simulink model "Inputs_Cond"  (Simulink 7.9)
settings: Solver=FixedStepDiscrete  StartTime=0.0  StopTime=10  RelTol=1e-3  SampleTimeConstraint=STIndependent
PreLoadFcn:
  | Input_Conditioning_selfinit
CloseFcn:
  | rtwprivate ssgencode ModelCloseRequest ADL
settings Model: MinMaxOverflowLogging=ForceOff  Creator=fguerin  LastModifiedBy=klindqvi  CovMetricSettings=dce  CovHTMLOptions=-aTS=1 -bRG=1 -bTC=1 -hTR=0 -nFC=0 -scm=1 -bcm=1 -xEv=0  CovHtmlReporting=off  covSaveCumulativeToWorkspaceVar=off  CovSaveSingleToWorkspaceVar=off  CovModelRefEnable=off  CovExternalEMLEnable=on
settings DataIOCC: ExternalInput=[t,u]  LimitDataPoints=off  SaveOutput=off  DSMLogging=off  SaveTime=off  SignalLoggingName=logsOut
settings OptimizationCC: InlineParams=on  InlineInvariantSignals=on  EnhancedBackFolding=on  ZeroExternalMemoryAtStartup=off  ZeroInternalMemoryAtStartup=off  EfficientFloat2IntCast=on  OptimizeModelRefInitCode=on  LifeSpan=1
settings DebuggingCC: ReadBeforeWriteMsg=EnableAllAsError  WriteAfterWriteMsg=EnableAllAsError  WriteAfterReadMsg=EnableAllAsError  AlgebraicLoopMsg=error  ArtificialAlgebraicLoopMsg=error  SaveWithDisabledLinksMsg=error  SaveWithParameterizedLinksMsg=error  CheckExecutionContextPreStartOutputMsg=on  CheckExecutionContextRuntimeOutputMsg=on  BlockPriorityViolationMsg=error  SolverPrmCheckMsg=error  MultiTaskCondExecSysMsg=warning  MultiTaskRateTransMsg=warning  IntegerOverflowMsg=none  ParameterUnderflowMsg=error  ParameterPrecisionLossMsg=error  ParameterTunabilityLossMsg=error  UnderSpecifiedDataTypeMsg=warning  UnnecessaryDatatypeConvMsg=warning  VectorMatrixConversionMsg=error  SignalLabelMismatchMsg=warning  SFcnCompatibilityMsg=error  BusObjectLabelMismatch=error  RootOutportRequireBusObject=error  AssertControl=DisableAll  ModelReferenceIOMsg=error  ModelReferenceIOMismatchMessage=error  ModelReferenceCSMismatchMessage=warning  UnknownTsInhSupMsg=error  ModelReferenceDataLoggingMessage=error  ModelReferenceSymbolNameMessage=none  StrictBusMsg=ErrorOnBusTreatedAsVector
settings HardwareCC: ProdLargestAtomicInteger=Long  ProdLargestAtomicFloat=Double  ProdIntDivRoundTo=Zero  ProdEndianess=BigEndian  ProdHWDeviceType=Freescale->MPC5500
settings ModelReferenceCC: ModelReferenceNumInstancesAllowed=Single
settings SFSimCC: SimParseCustomCode=off
settings RTWCC: SystemTargetFile=ert.tlc  TemplateMakefile=ert_default_tmf  Description=Embedded Coder  GenerateReport=on  RTWVerbose=off  ProcessScript=ert_make_rtw_hook  IncludeHyperlinkInReport=on  LaunchReport=on  GenerateTraceInfo=on  GenerateTraceReport=on  GenerateTraceReportSl=on  GenerateTraceReportSf=on  GenerateTraceReportEml=on  GenerateCodeMetricsReport=on
settings MATStruct: className=rtw.pil.Bullseye  argsAllComponents=[]  excludedModels=[]  includeReferencedModels=off  includeTopModel=on  enabled=on
settings CodeAppCC: ForceParamTrailComments=on  IgnoreCustomStorageClasses=off  IgnoreTestpoints=on  MangleLength=4  InlinedPrmAccess=Macros  ReqsInCode=on
settings ERTTargetCC: CodeReplacementLibrary=ANSI_C  MultiwordLength=2048  SupportAbsoluteTime=off  SupportNonFinite=off  SupportComplex=off  PortableWordSizes=on  InlinedParameterPlacement=NonHierarchical  ERTCustomFileTemplate=example_file_process.tlc  ConvertIfToSwitch=off  SuppressUnreachableDefaultCases=off
settings ConfigComp: Description=Design Verifier Custom Configuration Component  DVMaxProcessTime=600  DVDisplayUnsatisfiableObjectives=on  DVAutomaticStubbing=off  DVOutputDir=C:\Work\Data\Pilots\P_PSA_ECoder_BenchMark_LaGarenne\source9b\deliverable\trunk\demos\VnV_example\Projects\ADL_Project/Simulink_Test_Generation/ADL_Sim  DVModelCoverageObjectives=MCDC  DVTestSuiteOptimization=CombinedObjectives  DVDataFileName=./Tests/$ModelName$_sldvdata  DVSaveHarnessModel=on  DVHarnessModelFileName=./Tests/$ModelName$_testHarness  DVModelReferenceHarness=on  DVSaveReport=on  DVReportFileName=ADL_Sim_SLDV.html

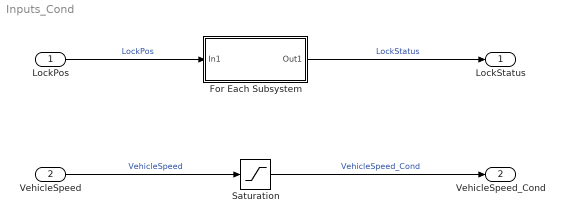
== system Inputs_Cond ==
  LockPos : Inport  OutDataTypeStr=fixdt('sfix16_Sp01')  PortDimensions=2
  VehicleSpeed : Inport  Port=2  OutDataTypeStr=single  PortDimensions=1
  For Each Subsystem : Subsystem  TreatAsAtomicUnit=on
  Saturation : Saturate  UpperLimit=350  LowerLimit=-50
  LockStatus : Outport  OutDataTypeStr=Enum: ActuatorStatus  PortDimensions=2
  VehicleSpeed_Cond : Outport  Port=2  OutDataTypeStr=single  PortDimensions=1
  wires:
  LockPos/1 -> For Each Subsystem/1(In1)  "LockPos"
  For Each Subsystem/1(Out1) -> LockStatus/1  "LockStatus"
  Saturation/1 -> VehicleSpeed_Cond/1  "VehicleSpeed_Cond"
  VehicleSpeed/1 -> Saturation/1  "VehicleSpeed"

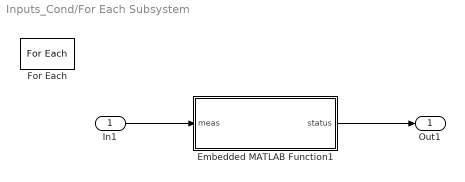
== system Inputs_Cond/For Each Subsystem ==
  In1 : Inport  Partition=on  PartitionDimension=1  PartitionWidth=1
  Embedded MATLAB Function1 : MATLAB Function  TreatAsAtomicUnit=on
  For Each : ForEach  DisableCoverage=on  IndexMode=One-based
  Out1 : Outport  ConcatenationDimension=1
  wires:
  Embedded MATLAB Function1/1(status) -> Out1/1
  In1/1 -> Embedded MATLAB Function1/1(meas)

== matlab function For Each Subsystem/Embedded MATLAB Function1 ==
  data: meas input double size=1; status output Enum: ActuatorStatus size=1
function status = getStatus(meas)
%#eml

if meas <= 1 %lockDoor_unlockPosition
    status = ActuatorStatus.UNLOCK_POS;
elseif meas >= 4 %lockDoor_lockPosition
    status = ActuatorStatus.LOCK_POS;
else
    status = ActuatorStatus.UNDETERMINED;
end
